simulink model "adaptivev2"  (R2024a)
settings: Solver=VariableStepAuto  StartTime=0.0  StopTime=2000  FixedStep=1E-4  MaxStep=1e-4  RelTol=1e-3
undefined symbols (not defined in the file or in its folder): estimator, initial_1
settings Model: Creator=b_ant  LastModifiedBy=b_ant
settings SolverCC: ZeroCrossAlgorithm=Adaptive  SolverResetMethod=Robust
settings DebuggingCC: IgnoredZcDiagnostic=none

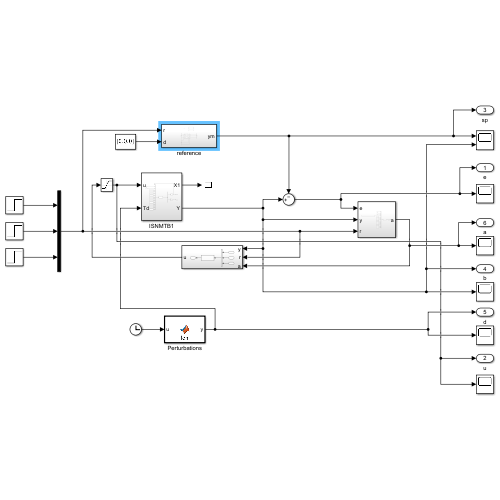
[thumbnail: Simulink's stored preview of the top-level diagram]
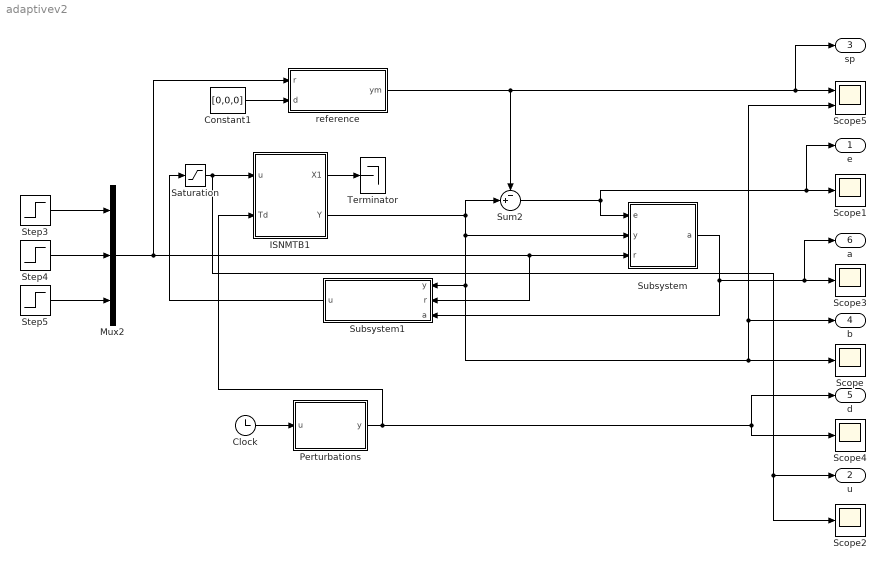
== system adaptivev2 ==
  Clock : Clock
      settings: Decimation=1000
  Constant1 : Constant  Value=[0,0,0]
  ISNMTB1 : Subsystem
  Mux2 : Mux  Inputs=3
  Perturbations : MATLAB Function  TreatAsAtomicUnit=on
  Saturation : Saturate  UpperLimit=[50,50,50]'  LowerLimit=-[50,50,50]'
  Scope{,1..4} (5 alike) : Scope
  Scope5 : Scope  NumInputPorts=2
  Step3 : Step  Time=0.1  After=0  SampleTime=0
  Step4 : Step  Time=0.1  After=0  SampleTime=0
  Step5 : Step  Time=0.1  After=0  SampleTime=0
  Subsystem : Subsystem
  Subsystem1 : Subsystem
  Sum2 : Sum  Inputs=-+|
  Terminator : Terminator
  reference : Subsystem
  e : Outport
  u : Outport  Port=2
  sp : Outport  Port=3
  b : Outport  Port=4
  d : Outport  Port=5
  a : Outport  Port=6
  wires:
  Clock/1 -> Perturbations/1(u)
  reference/1(ym) -> Sum2/1, Scope5/1, sp/1
  Step4/1 -> Mux2/2
  Step5/1 -> Mux2/3
  Step3/1 -> Mux2/1
  Mux2/1 -> reference/1(r), Subsystem1/2(r), Subsystem/3(r)
  Subsystem/1(a) -> Subsystem1/3(a), a/1, Scope3/1
  Sum2/1 -> Subsystem/1(e), e/1, Scope1/1
  ISNMTB1/2(Y) -> Subsystem/2(y), Scope/1, Scope5/2, b/1, Subsystem1/1(y), Sum2/2
  Constant1/1 -> reference/2(d)
  Perturbations/1(y) -> ISNMTB1/2(Td), d/1, Scope4/1
  ISNMTB1/1(X1) -> Terminator/1
  Subsystem1/1(u) -> Saturation/1
  Saturation/1 -> ISNMTB1/1(u), u/1, Scope2/1

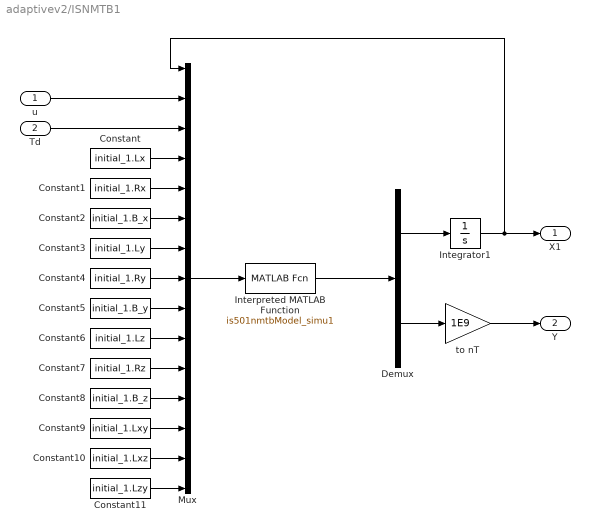
== system adaptivev2/ISNMTB1 ==
  u : Inport
  Td : Inport  Port=2
  Constant : Constant  Value=initial_1.Lx
  Constant1 : Constant  Value=initial_1.Rx
  Constant10 : Constant  Value=initial_1.Lxz
  Constant11 : Constant  Value=initial_1.Lzy
  Constant2 : Constant  Value=initial_1.B_x
  Constant3 : Constant  Value=initial_1.Ly
  Constant4 : Constant  Value=initial_1.Ry
  Constant5 : Constant  Value=initial_1.B_y
  Constant6 : Constant  Value=initial_1.Lz
  Constant7 : Constant  Value=initial_1.Rz
  Constant8 : Constant  Value=initial_1.B_z
  Constant9 : Constant  Value=initial_1.Lxy
  Demux : Demux  Outputs=2
  Integrator1 : Integrator  InitialCondition=[0,0,0]'
  Interpreted MATLAB Function : MATLABFcn  MATLABFcn=is501nmtbModel_simu1  OutputDimensions=6
  Mux : Mux  Inputs=15
  to nT : Gain  Gain=1E9
  X1 : Outport
  Y : Outport  Port=2
  wires:
  Mux/1 -> Interpreted MATLAB Function/1
  u/1 -> Mux/2
  Td/1 -> Mux/3
  Constant/1 -> Mux/4
  Constant1/1 -> Mux/5
  Constant2/1 -> Mux/6
  Constant3/1 -> Mux/7
  Constant4/1 -> Mux/8
  Constant5/1 -> Mux/9
  Constant6/1 -> Mux/10
  Constant7/1 -> Mux/11
  Constant8/1 -> Mux/12
  Constant9/1 -> Mux/13
  Constant10/1 -> Mux/14
  Constant11/1 -> Mux/15
  Interpreted MATLAB Function/1 -> Demux/1
  Demux/1 -> Integrator1/1
  Demux/2 -> to nT/1
  to nT/1 -> Y/1
  Integrator1/1 -> Mux/1, X1/1

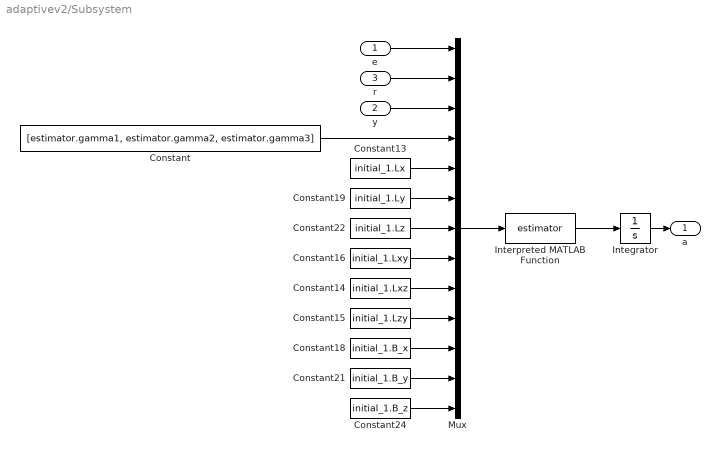
== system adaptivev2/Subsystem ==
  e : Inport
  y : Inport  Port=2
  r : Inport  Port=3
  Constant : Constant  Value=[estimator.gamma1, estimator.gamma2, estimator.gamma3]
  Constant13 : Constant  Value=initial_1.Lx
  Constant14 : Constant  Value=initial_1.Lxz
  Constant15 : Constant  Value=initial_1.Lzy
  Constant16 : Constant  Value=initial_1.Lxy
  Constant18 : Constant  Value=initial_1.B_x
  Constant19 : Constant  Value=initial_1.Ly
  Constant21 : Constant  Value=initial_1.B_y
  Constant22 : Constant  Value=initial_1.Lz
  Constant24 : Constant  Value=initial_1.B_z
  Integrator : Integrator  InitialCondition=[0,0,0,0,0,0]
  Interpreted MATLAB Function : MATLABFcn  MATLABFcn=estimator  OutputDimensions=6
  Mux : Mux  Inputs=13
  a : Outport
  wires:
  Constant21/1 -> Mux/12
  Constant19/1 -> Mux/6
  Constant/1 -> Mux/4
  Constant16/1 -> Mux/8
  Constant18/1 -> Mux/11
  y/1 -> Mux/3
  Constant24/1 -> Mux/13
  Constant13/1 -> Mux/5
  Constant22/1 -> Mux/7
  Interpreted MATLAB Function/1 -> Integrator/1
  r/1 -> Mux/2
  Constant14/1 -> Mux/9
  Constant15/1 -> Mux/10
  Mux/1 -> Interpreted MATLAB Function/1
  e/1 -> Mux/1
  Integrator/1 -> a/1

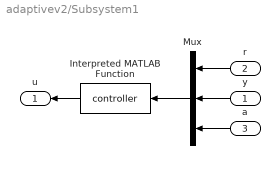
== system adaptivev2/Subsystem1 ==
  y : Inport
  r : Inport  Port=2
  a : Inport  Port=3
  Interpreted MATLAB Function : MATLABFcn  MATLABFcn=controller
  Mux : Mux  Inputs=3
  u : Outport
  wires:
  Mux/1 -> Interpreted MATLAB Function/1
  Interpreted MATLAB Function/1 -> u/1
  a/1 -> Mux/3
  r/1 -> Mux/1
  y/1 -> Mux/2

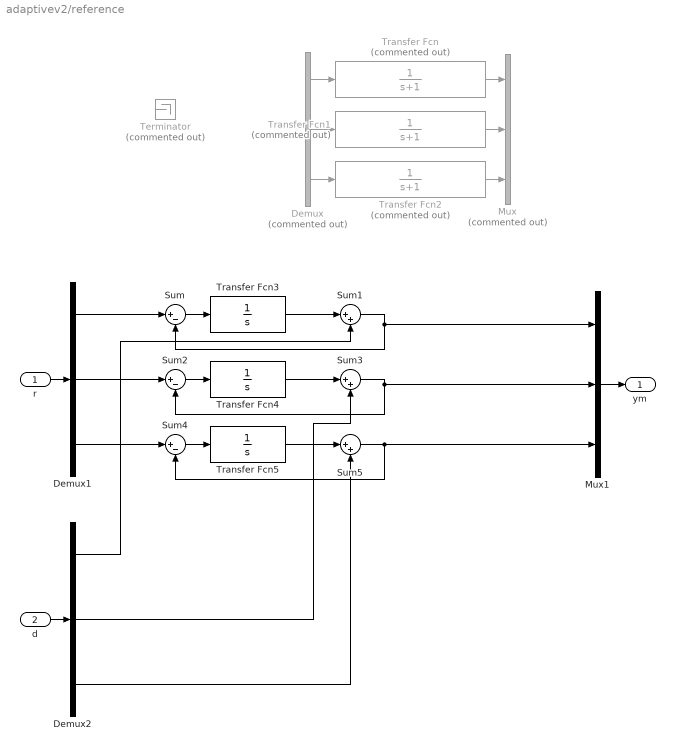
== system adaptivev2/reference ==
  r : Inport
  d : Inport  Port=2
  Demux : Demux  Commented=on  Outputs=3
  Demux1 : Demux  Outputs=3
  Demux2 : Demux  Outputs=3
  Mux : Mux  Commented=on  Inputs=3
  Mux1 : Mux  Inputs=3
  Sum : Sum  Inputs=|+-
  Sum1 : Sum  Inputs=|++
  Sum2 : Sum  Inputs=|+-
  Sum3 : Sum  Inputs=|++
  Sum4 : Sum  Inputs=|+-
  Sum5 : Sum  Inputs=|++
  Terminator : Terminator  Commented=on
  Transfer Fcn : TransferFcn  Commented=on  Numerator=1  Denominator=[1 1]
  Transfer Fcn1 : TransferFcn  Commented=on  Numerator=1  Denominator=[1 1]
  Transfer Fcn2 : TransferFcn  Commented=on  Numerator=1  Denominator=[1 1]
  Transfer Fcn3 : TransferFcn  Numerator=1  Denominator=[1 0]
  Transfer Fcn4 : TransferFcn  Numerator=1  Denominator=[1 0]
  Transfer Fcn5 : TransferFcn  Numerator=1  Denominator=[1 0]
  ym : Outport
  wires:
  Demux/2 -> Transfer Fcn1/1
  Transfer Fcn/1 -> Mux/1
  Demux/1 -> Transfer Fcn/1
  Demux/3 -> Transfer Fcn2/1
  Transfer Fcn1/1 -> Mux/2
  Transfer Fcn2/1 -> Mux/3
  Sum5/1 -> Sum4/2, Mux1/3
  Sum3/1 -> Sum2/2, Mux1/2
  Demux1/1 -> Sum/1
  Sum/1 -> Transfer Fcn3/1
  Transfer Fcn3/1 -> Sum1/1
  Sum1/1 -> Sum/2, Mux1/1
  Sum2/1 -> Transfer Fcn4/1
  Transfer Fcn4/1 -> Sum3/1
  Sum4/1 -> Transfer Fcn5/1
  Transfer Fcn5/1 -> Sum5/1
  Demux1/2 -> Sum2/1
  Demux1/3 -> Sum4/1
  Demux2/1 -> Sum1/2
  Demux2/2 -> Sum3/2
  Demux2/3 -> Sum5/2
  d/1 -> Demux2/1
  Mux1/1 -> ym/1
  r/1 -> Demux1/1

== matlab function adaptivev2/Perturbations ==
  data: u input; y output
function y = fcn(u)
y= [2.522*sin(2*pi*4.788E-3*u)+3.249E04;
   -5.174*sin(2*pi*7.481E-3*u)-2.265E04;
    3.359*sin(2*pi*8.378E-3*u)+3.655E04]*1E-9;
end
